simulink model "BeagleBone_Roll_Pitch_R_Kalman_Tuning"  (R2024a)
settings: Solver=FixedStepAuto  StartTime=0.0  StopTime=inf  RelTol=1e-3  EnableMultiTasking=on
libraries: simulink_extras x1, bbblueSensorLib x1
settings Model: ExtModeTrigDuration=100  Creator=eduar  LastModifiedBy=eduar
settings SolverCC: PositivePriorityOrder=on
settings OptimizationCC: EnhancedBackFolding=on  PassReuseOutputArgsAs=Individual arguments  ZeroExternalMemoryAtStartup=off  ZeroInternalMemoryAtStartup=off  MaxStackSize=64  OptimizeBlockOrder=speed  DifferentSizesBufferReuse=on  OptimizationCustomize=off  EfficientTunableParamExpr=on
settings DebuggingCC: ParameterTunabilityLossMsg=error
settings HardwareCC: ProdBitPerPointer=32  ProdBitPerSizeT=32  ProdBitPerPtrDiffT=32  ProdLargestAtomicInteger=Long  ProdLargestAtomicFloat=Double  ProdWordSize=32  ProdHWDeviceType=ARM Compatible->ARM Cortex
settings SFSimCC: MATLABDynamicMemAlloc=off
settings RTWCC: Description=Embedded Coder  SystemTargetFile=ert.tlc  HardwareBoard=BeagleBone Blue  TLCOptions="-aInlineSetEventsForThisBaseRateFcn=TLC_FALSE -aSuppressMultiTaskScheduler=TLC_FALSE  -aRateBasedStepFcn=0"  TemplateMakefile=ert_default_tmf  Toolchain=GNU GCC BeagleBone Blue
settings CodeAppCC: ForceParamTrailComments=on  IgnoreCustomStorageClasses=off  OperatorAnnotations=on  SimulinkDataObjDesc=on  SFDataObjDesc=on  InsertBlockDesc=on
settings ERTTargetCC: SupportVariableSizeSignals=on

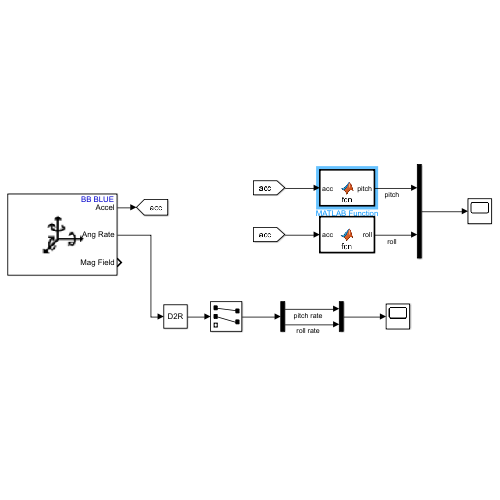
[thumbnail: Simulink's stored preview of the top-level diagram]
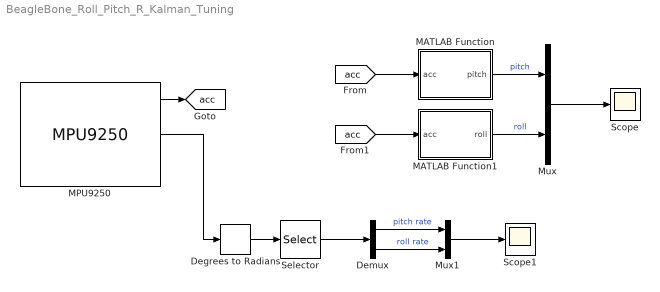
== system BeagleBone_Roll_Pitch_R_Kalman_Tuning ==
  Degrees to Radians : simulink_extras/Transformations/Degrees to Radians
  Demux : Demux  Outputs=2
  MATLAB Function : MATLAB Function  TreatAsAtomicUnit=on
  MATLAB Function1 : MATLAB Function  TreatAsAtomicUnit=on
  MPU9250 : bbblueSensorLib/MPU9250  OperationMode=DMP  Accel=on  AngularRate=on  Ak8963Field=on  EulerAngles=off  Quat=off  AccelRange=2G  Acceldlpf=1  GyroRange=250 dps  Gyrodlpf=1  DmpOdr=200 Hz  SampleTime=0.1
  Mux : Mux  Inputs=2
  Mux1 : Mux  Inputs=2
  Scope : Scope
  Scope1 : Scope
  Selector : Selector  InputPortWidth=3  IndexOptions=Index vector (dialog)  Indices=[1 2]  OutputSizes=1
  tag scope: acc=global
  wires:
  MATLAB Function1/1(roll) -> Mux/2  "roll"
  MATLAB Function/1(pitch) -> Mux/1  "pitch"
  Mux/1 -> Scope/1
  MPU9250/1 -> [acc]
  [acc] -> MATLAB Function/1(acc)
  [acc] -> MATLAB Function1/1(acc)
  MPU9250/2 -> Degrees to Radians/1
  Selector/1 -> Demux/1
  Demux/1 -> Mux1/1  "pitch rate"
  Demux/2 -> Mux1/2  "roll rate"
  Mux1/1 -> Scope1/1
  Degrees to Radians/1 -> Selector/1

== matlab function BeagleBone_Roll_Pitch_R_Kalman_Tuning/MATLAB Function ==
  data: acc input; pitch output
function pitch = fcn(acc)

acc_x = acc(1); % declaring accel x
acc_z = acc(3); % declaring acceleromoter z

pitch = atan(acc_x/acc_z);

end

== matlab function BeagleBone_Roll_Pitch_R_Kalman_Tuning/MATLAB Function1 ==
  data: acc input; roll output
function roll = fcn(acc)

acc_y = acc(2); % declaring accel x
acc_z = acc(3); % declaring acceleromoter z

roll = atan(acc_y/acc_z);

end
